simulink model "SPWM_3ph"  (R2014b)
settings: Solver=ode45  StartTime=0.0  StopTime=1  RelTol=1e-3
libraries: powerlib x10, powerlib_meascontrol x2
settings Model: Creator=amir  LastModifiedBy=amir_p
settings DebuggingCC: UnderspecifiedInitializationDetection=Classic  MergeDetectMultiDrivingBlocksExec=none  StateNameClashWarn=warning

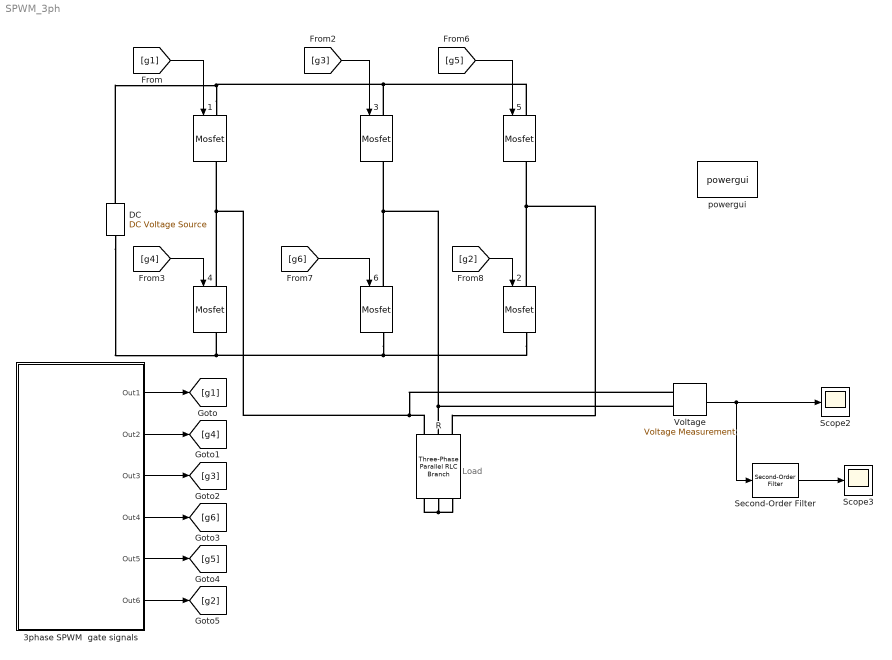
== system SPWM_3ph ==
  note: Load
  " 3phase SPWM  gate signals" : Subsystem
  {1..6} (6 alike) : powerlib/Power Electronics/Mosfet  Ron=0.1  Lon=0  Rd=0.01  Vfd=0  IC=0  Rs=1e5  Cs=inf  Measurements=on
  "DC  " : powerlib/Electrical Sources/DC Voltage Source  Amplitude=380*sqrt(2)  Measurements=None
  R : powerlib/Elements/Three-Phase Parallel RLC Branch  LConnTagsString=A|B|C  RConnTagsString=A|B|C  BranchType=R  Resistance=100  Inductance=1e-3  Capacitance=1e-6  Measurements=None
  Scope2 : Scope
      settings: SaveName=V
  Scope3 : Scope
      settings: YMin=-110  YMax=110  SaveName=Vfilter
  Second-Order Filter : powerlib_meascontrol/Filters/Second-Order Filter  FilterType=Lowpass  Fo=50  Zeta=0.707  Ts=0  Initialize=on  Vac_Init="[0,  0,  50]"  Vdc_Init=0  PlotResponse=off  FreqRange=[0, 500, 1]
  "Voltage " : powerlib/Measurements/Voltage Measurement  PhasorSimulation=off  OutputType=Complex  PSBequivalent=0
  powergui : powerlib/powergui  Priority=1  SimulationMode=Discrete  SolverType=Tustin  SampleTime=50e-6  frequency=60  SPID=off  DisableSnubberDevices=on  DisableRonSwitches=on  DisableVfSwitches=on  SwTol=0  DisplayEquations=on  Interpol=off  methode=off  Ts=0  frequencyindice=0  Pbase=100e6  ErrMax=1e-4  Iterations=50  UnitsV=kV  UnitsW=MW  FunctionMessages=off  echomessages=off  HookPort=off  EnableUseOfTLC=off  x0status=blocks  RestoreLinks=warning  ResistiveCurrentMeasurement=off  Frange=[0:2:500]  Ylog=off  Xlog=on  ShowGrid=off  save=off  variable=ZData  structure=V3h  ZoomFFT=off  StartTime=0.1  cycles=1  DisplayStyle=2  fundamental=50  FreqAxis=off  MaxFrequency=3000  frequencyindicesteady=1  RmsSteady=1  display=off
  wires:
  [g1] -> 1/1
  [g2] -> 2/1
  [g3] -> 3/1
  [g4] -> 4/1
  [g5] -> 5/1
  [g6] -> 6/1
  "Voltage "/1 -> Scope2/1, Second-Order Filter/1
  Second-Order Filter/1 -> Scope3/1
  " 3phase SPWM  gate signals"/1(Out1) -> [g1]
  " 3phase SPWM  gate signals"/2(Out2) -> [g4]
  " 3phase SPWM  gate signals"/3(Out3) -> [g3]
  " 3phase SPWM  gate signals"/4(Out4) -> [g6]
  " 3phase SPWM  gate signals"/5(Out5) -> [g5]
  " 3phase SPWM  gate signals"/6(Out6) -> [g2]
  connections:
  2/RConn1 -- 6/RConn1 -- "DC  "/LConn1 -- 4/RConn1
  1/RConn1 -- 4/LConn1 -- "Voltage "/LConn1 -- R/LConn1
  3/RConn1 -- 6/LConn1 -- R/LConn2 -- "Voltage "/LConn2
  5/RConn1 -- 2/LConn1 -- R/LConn3
  1/LConn1 -- "DC  "/RConn1 -- 5/LConn1 -- 3/LConn1
  R/RConn1 -- R/RConn3 -- R/RConn2

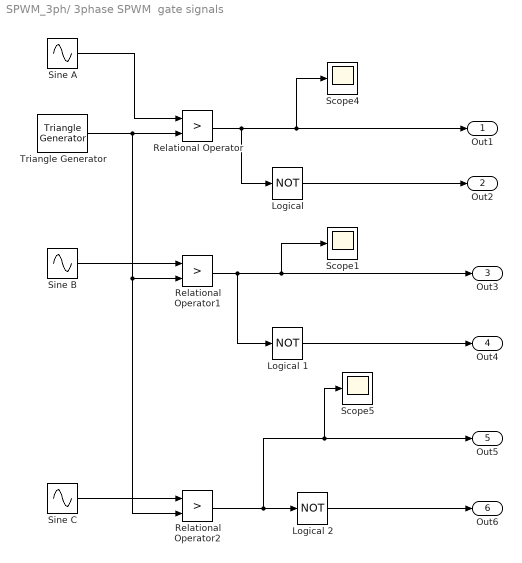
== system SPWM_3ph/ 3phase SPWM  gate signals ==
  "Logical " : Logic  Operator=NOT  AllPortsSameDT=off  OutDataTypeStr=boolean
  Logical 1 : Logic  Operator=NOT  AllPortsSameDT=off  OutDataTypeStr=boolean
  Logical 2 : Logic  Operator=NOT  AllPortsSameDT=off  OutDataTypeStr=boolean
  Relational Operator : RelationalOperator  Operator=>  OutDataTypeStr=boolean
  Relational Operator1 : RelationalOperator  Operator=>  OutDataTypeStr=boolean
  Relational Operator2 : RelationalOperator  Operator=>  OutDataTypeStr=boolean
  Scope1 : Scope
      settings: SaveName=V2
  Scope4 : Scope
      settings: SaveName=V1
  Scope5 : Scope
      settings: SaveName=V3
  Sine A : Sin  Frequency=2*pi*50  SampleTime=0
  Sine B : Sin  Frequency=2*pi*50  Phase=-2*pi/3  SampleTime=0
  Sine C : Sin  Frequency=2*pi*50  Phase=-4*pi/3  SampleTime=0
  Triangle Generator : powerlib_meascontrol/Pulse & Signal Generators/Triangle Generator  Freq=1e3  Phase=0  Ts=0
  Out1 : Outport
  Out2 : Outport  Port=2
  Out3 : Outport  Port=3
  Out4 : Outport  Port=4
  Out5 : Outport  Port=5
  Out6 : Outport  Port=6
  wires:
  Sine C/1 -> Relational Operator2/1
  Sine B/1 -> Relational Operator1/1
  Sine A/1 -> Relational Operator/1
  Triangle Generator/1 -> Relational Operator2/2, Relational Operator1/2, Relational Operator/2
  Relational Operator/1 -> "Logical "/1, Out1/1, Scope4/1
  Relational Operator1/1 -> Logical 1/1, Out3/1, Scope1/1
  Logical 2/1 -> Out6/1
  Logical 1/1 -> Out4/1
  Relational Operator2/1 -> Out5/1, Scope5/1, Logical 2/1
  "Logical "/1 -> Out2/1
